simulink library "flaglib"  (R2018b)
settings: Solver=VariableStepAuto  StartTime=0.0  StopTime=10.0  RelTol=1e-3
settings Model: Creator=billg  LastModifiedBy=billg

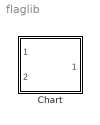
== system flaglib ==
  Chart : Stateflow chart  TreatAsAtomicUnit=on

== stateflow chart flaglib/Chart ==
  state Init
    entry:
    flagMotor = 0;
  state Raising
    entry:
    flagMotor = 20;
  state StopRaising
    entry:
    flagMotor = 0;
  state StopLowering
    entry:
    flagMotor = 0;
  state StartLowering
    entry:
    flagMotor = -20;
  (default) -> Init
  Raising -> StopRaising : [encoder >= 90]
  Init -> Raising : [button == 1]
  StopLowering -> Raising : [button == 1]
  StopRaising -> StartLowering : [button == 1]
  StartLowering -> StopLowering : [encoder <= 0]
  data: encoder input; flagMotor output; button input
